simulink model "case4"  (R2024b)
settings: Solver=FixedStepAuto  StartTime=0  StopTime=1  FixedStep=1e-7  RelTol=1e-3
values from neighbouring files (symbols this model uses):
  SG_D_1_D = 0.01056    [IEEE9_case_parameters.m]    (also in case1_parameters.m; case2_parameters.m; case3_parameters.m; case4_parameters.m)
  SG_D_1_EnableSaturation = 0    [IEEE9_case_parameters.m]    (also in case1_parameters.m; case2_parameters.m; case3_parameters.m; case4_parameters.m)
  SG_D_1_f0 = 60    [IEEE9_case_parameters.m]    (also in case1_parameters.m; case2_parameters.m; case3_parameters.m; case4_parameters.m)
  SG_D_1_H = 7.5    [IEEE9_case_parameters.m]    (also in case1_parameters.m; case2_parameters.m; case3_parameters.m; case4_parameters.m)
  SG_D_1_K_A = 20    [IEEE9_case_parameters.m]    (also in case1_parameters.m; case2_parameters.m; case3_parameters.m; case4_parameters.m)
  SG_D_1_K_E = 1.000000e+1    (= 10)    [IEEE9_case_parameters.m]    (also in case1_parameters.m; case2_parameters.m; case3_parameters.m; case4_parameters.m)
  SG_D_1_K_F = 2.363    [IEEE9_case_parameters.m]    (also in case1_parameters.m; case2_parameters.m; case3_parameters.m; case4_parameters.m)
  SG_D_1_K_s = 0.5    [IEEE9_case_parameters.m]    (also in case1_parameters.m = 5; case2_parameters.m = 5; case3_parameters.m = 5; case4_parameters.m = 5)
  SG_D_1_R_a = 0.001088    [IEEE9_case_parameters.m]    (also in case1_parameters.m; case2_parameters.m; case3_parameters.m; case4_parameters.m)
  SG_D_1_S_A = 1    [IEEE9_case_parameters.m]    (also in case1_parameters.m; case2_parameters.m; case3_parameters.m; case4_parameters.m)
  SG_D_1_S_B = 0.103    [IEEE9_case_parameters.m]    (also in case1_parameters.m; case2_parameters.m; case3_parameters.m; case4_parameters.m)
  SG_D_1_S_N = 10.659857    [IEEE9_case_parameters.m]    (also in case1_parameters.m; case2_parameters.m; case3_parameters.m; case4_parameters.m)
  SG_D_1_SpeedPara = 200    [IEEE9_case_parameters.m]    (also in case1_parameters.m; case2_parameters.m; case3_parameters.m; case4_parameters.m)
  SG_D_1_T_0 = 0.720173    [IEEE9_case_parameters.m]    (also in case1_parameters.m = 0.755522; case2_parameters.m = 0.808931; case3_parameters.m = 0.869402; case4_parameters.m = 0.729316)
  SG_D_1_T_1 = 0.3    [IEEE9_case_parameters.m]    (also in case1_parameters.m; case2_parameters.m; case3_parameters.m; case4_parameters.m)
  SG_D_1_T_2 = 0.05    [IEEE9_case_parameters.m]    (also in case1_parameters.m; case2_parameters.m; case3_parameters.m; case4_parameters.m)
  SG_D_1_T_3 = 0.02    [IEEE9_case_parameters.m]    (also in case1_parameters.m; case2_parameters.m; case3_parameters.m; case4_parameters.m)
  SG_D_1_T_4 = 0.005    [IEEE9_case_parameters.m]    (also in case1_parameters.m; case2_parameters.m; case3_parameters.m; case4_parameters.m)
  SG_D_1_T_A = 0.02    [IEEE9_case_parameters.m]    (also in case1_parameters.m; case2_parameters.m; case3_parameters.m; case4_parameters.m)
  SG_D_1_T_dd = 8.000000e+0    (= 8)    [IEEE9_case_parameters.m]    (also in case1_parameters.m; case2_parameters.m; case3_parameters.m; case4_parameters.m)
  SG_D_1_T_ddd = 0.04    [IEEE9_case_parameters.m]    (also in case1_parameters.m; case2_parameters.m; case3_parameters.m; case4_parameters.m)
  SG_D_1_T_E = 0.314    [IEEE9_case_parameters.m]    (also in case1_parameters.m; case2_parameters.m; case3_parameters.m; case4_parameters.m)
  SG_D_1_T_F = 0.35    [IEEE9_case_parameters.m]    (also in case1_parameters.m; case2_parameters.m; case3_parameters.m; case4_parameters.m)
  SG_D_1_T_qd = 0.8    [IEEE9_case_parameters.m]    (also in case1_parameters.m; case2_parameters.m; case3_parameters.m; case4_parameters.m)
  SG_D_1_T_qdd = 0.02    [IEEE9_case_parameters.m]    (also in case1_parameters.m; case2_parameters.m; case3_parameters.m; case4_parameters.m)
  SG_D_1_T_speed = 0.1    [IEEE9_case_parameters.m]    (also in case1_parameters.m = 200; case2_parameters.m = 200; case3_parameters.m = 200; case4_parameters.m = 200)
  SG_D_1_T_w = 0.5    [IEEE9_case_parameters.m]    (also in case1_parameters.m; case2_parameters.m; case3_parameters.m; case4_parameters.m)
  SG_D_1_V_ref = 1.990276    [IEEE9_case_parameters.m]    (also in case1_parameters.m = 2.042296; case2_parameters.m = 2.051388; case3_parameters.m = 2.089584; case4_parameters.m = 2.01845)
  SG_D_1_w_ref = 376.991118    [IEEE9_case_parameters.m]    (also in case1_parameters.m; case2_parameters.m; case3_parameters.m; case4_parameters.m)
  SG_D_1_wb = 6.000000e+1    (= 60)    [IEEE9_case_parameters.m]    (also in case1_parameters.m; case2_parameters.m; case3_parameters.m; case4_parameters.m)
  SG_D_1_x_d = 1.9    [IEEE9_case_parameters.m]    (also in case1_parameters.m; case2_parameters.m; case3_parameters.m; case4_parameters.m)
  SG_D_1_x_dd = 0.302    [IEEE9_case_parameters.m]    (also in case1_parameters.m; case2_parameters.m; case3_parameters.m; case4_parameters.m)
  SG_D_1_x_ddd = 0.204    [IEEE9_case_parameters.m]    (also in case1_parameters.m; case2_parameters.m; case3_parameters.m; case4_parameters.m)
  SG_D_1_x_l = 0.05    [IEEE9_case_parameters.m]    (also in case1_parameters.m; case2_parameters.m; case3_parameters.m; case4_parameters.m)
  SG_D_1_x_q = 1.3    [IEEE9_case_parameters.m]    (also in case1_parameters.m; case2_parameters.m; case3_parameters.m; case4_parameters.m)
  SG_D_1_x_qd = 0.5    [IEEE9_case_parameters.m]    (also in case1_parameters.m; case2_parameters.m; case3_parameters.m; case4_parameters.m)
  SG_D_1_x_qdd = 0.3    [IEEE9_case_parameters.m]    (also in case1_parameters.m; case2_parameters.m; case3_parameters.m; case4_parameters.m)
  SG_D_2_D = 0.02    [IEEE9_case_parameters.m]    (also in case1_parameters.m; case2_parameters.m; case3_parameters.m; case4_parameters.m)
  SG_D_2_EnableSaturation = 0    [IEEE9_case_parameters.m]    (also in case1_parameters.m; case2_parameters.m; case3_parameters.m; case4_parameters.m)
  SG_D_2_f0 = 60    [IEEE9_case_parameters.m]    (also in case1_parameters.m; case2_parameters.m; case3_parameters.m; case4_parameters.m)
  SG_D_2_H = 8.000000e+0    (= 8)    [IEEE9_case_parameters.m]    (also in case1_parameters.m; case2_parameters.m; case3_parameters.m; case4_parameters.m)
  SG_D_2_K_A = 20    [IEEE9_case_parameters.m]    (also in case1_parameters.m; case2_parameters.m; case3_parameters.m; case4_parameters.m)
  SG_D_2_K_E = 1.000000e+1    (= 10)    [IEEE9_case_parameters.m]    (also in case1_parameters.m; case2_parameters.m; case3_parameters.m; case4_parameters.m)
  SG_D_2_K_F = 2.363    [IEEE9_case_parameters.m]    (also in case1_parameters.m; case2_parameters.m; case3_parameters.m; case4_parameters.m)
  SG_D_2_K_s = 0.5    [IEEE9_case_parameters.m]    (also in case1_parameters.m = 4; case2_parameters.m = 4; case3_parameters.m = 4; case4_parameters.m = 4)
  SG_D_2_R_a = 0.001088    [IEEE9_case_parameters.m]    (also in case1_parameters.m; case2_parameters.m; case3_parameters.m; case4_parameters.m)
  SG_D_2_S_A = 1    [IEEE9_case_parameters.m]    (also in case1_parameters.m; case2_parameters.m; case3_parameters.m; case4_parameters.m)
  SG_D_2_S_B = 0.103    [IEEE9_case_parameters.m]    (also in case1_parameters.m; case2_parameters.m; case3_parameters.m; case4_parameters.m)
  SG_D_2_S_N = 10.659857    [IEEE9_case_parameters.m]    (also in case1_parameters.m; case2_parameters.m; case3_parameters.m; case4_parameters.m)
  SG_D_2_SpeedPara = 200    [IEEE9_case_parameters.m]    (also in case1_parameters.m; case2_parameters.m; case3_parameters.m; case4_parameters.m)
  SG_D_2_T_0 = 1.632913    [IEEE9_case_parameters.m]    (also in case1_parameters.m = 1.632925; case2_parameters.m = 1.632915; case3_parameters.m = 1.632914; case4_parameters.m = 1.632927)
  SG_D_2_T_1 = 0.2    [IEEE9_case_parameters.m]    (also in case1_parameters.m; case2_parameters.m; case3_parameters.m; case4_parameters.m)
  SG_D_2_T_2 = 0.05    [IEEE9_case_parameters.m]    (also in case1_parameters.m; case2_parameters.m; case3_parameters.m; case4_parameters.m)
  SG_D_2_T_3 = 0.02    [IEEE9_case_parameters.m]    (also in case1_parameters.m; case2_parameters.m; case3_parameters.m; case4_parameters.m)
  SG_D_2_T_4 = 0.005    [IEEE9_case_parameters.m]    (also in case1_parameters.m; case2_parameters.m; case3_parameters.m; case4_parameters.m)
  SG_D_2_T_A = 0.02    [IEEE9_case_parameters.m]    (also in case1_parameters.m; case2_parameters.m; case3_parameters.m; case4_parameters.m)
  SG_D_2_T_dd = 7.9    [IEEE9_case_parameters.m]    (also in case1_parameters.m; case2_parameters.m; case3_parameters.m; case4_parameters.m)
  SG_D_2_T_ddd = 0.04    [IEEE9_case_parameters.m]    (also in case1_parameters.m; case2_parameters.m; case3_parameters.m; case4_parameters.m)
  SG_D_2_T_E = 0.314    [IEEE9_case_parameters.m]    (also in case1_parameters.m; case2_parameters.m; case3_parameters.m; case4_parameters.m)
  SG_D_2_T_F = 0.35    [IEEE9_case_parameters.m]    (also in case1_parameters.m; case2_parameters.m; case3_parameters.m; case4_parameters.m)
  SG_D_2_T_qd = 0.8    [IEEE9_case_parameters.m]    (also in case1_parameters.m; case2_parameters.m; case3_parameters.m; case4_parameters.m)
  SG_D_2_T_qdd = 0.015    [IEEE9_case_parameters.m]    (also in case1_parameters.m; case2_parameters.m; case3_parameters.m; case4_parameters.m)
  SG_D_2_T_speed = 0.1    [IEEE9_case_parameters.m]    (also in case1_parameters.m = 150; case2_parameters.m = 150; case3_parameters.m = 150; case4_parameters.m = 150)
  SG_D_2_T_w = 0.35    [IEEE9_case_parameters.m]    (also in case1_parameters.m; case2_parameters.m; case3_parameters.m; case4_parameters.m)
  SG_D_2_V_ref = 2.58547    [IEEE9_case_parameters.m]    (also in case1_parameters.m = 2.597896; case2_parameters.m = 2.587136; case3_parameters.m = 2.586042; case4_parameters.m = 2.599679)
  SG_D_2_w_ref = 376.991118    [IEEE9_case_parameters.m]    (also in case1_parameters.m; case2_parameters.m; case3_parameters.m; case4_parameters.m)
  SG_D_2_wb = 6.000000e+1    (= 60)    [IEEE9_case_parameters.m]    (also in case1_parameters.m; case2_parameters.m; case3_parameters.m; case4_parameters.m)
  SG_D_2_x_d = 1.8    [IEEE9_case_parameters.m]    (also in case1_parameters.m; case2_parameters.m; case3_parameters.m; case4_parameters.m)
  SG_D_2_x_dd = 0.302    [IEEE9_case_parameters.m]    (also in case1_parameters.m; case2_parameters.m; case3_parameters.m; case4_parameters.m)
  SG_D_2_x_ddd = 0.204    [IEEE9_case_parameters.m]    (also in case1_parameters.m; case2_parameters.m; case3_parameters.m; case4_parameters.m)
  SG_D_2_x_l = 0.05    [IEEE9_case_parameters.m]    (also in case1_parameters.m; case2_parameters.m; case3_parameters.m; case4_parameters.m)
  SG_D_2_x_q = 1.25    [IEEE9_case_parameters.m]    (also in case1_parameters.m; case2_parameters.m; case3_parameters.m; case4_parameters.m)
  SG_D_2_x_qd = 0.5    [IEEE9_case_parameters.m]    (also in case1_parameters.m; case2_parameters.m; case3_parameters.m; case4_parameters.m)
  SG_D_2_x_qdd = 0.3    [IEEE9_case_parameters.m]    (also in case1_parameters.m; case2_parameters.m; case3_parameters.m; case4_parameters.m)
  SG_D_3_D = 0.02    [IEEE9_case_parameters.m]    (also in case1_parameters.m; case2_parameters.m; case3_parameters.m; case4_parameters.m)
  SG_D_3_EnableSaturation = 0    [IEEE9_case_parameters.m]    (also in case1_parameters.m; case2_parameters.m; case3_parameters.m; case4_parameters.m)
  SG_D_3_f0 = 60    [IEEE9_case_parameters.m]    (also in case1_parameters.m; case2_parameters.m; case3_parameters.m; case4_parameters.m)
  SG_D_3_H = 7.7    [IEEE9_case_parameters.m]    (also in case1_parameters.m; case2_parameters.m; case3_parameters.m; case4_parameters.m)
  SG_D_3_K_A = 20    [IEEE9_case_parameters.m]    (also in case1_parameters.m; case2_parameters.m; case3_parameters.m; case4_parameters.m)
  SG_D_3_K_E = 1.000000e+1    (= 10)    [IEEE9_case_parameters.m]    (also in case1_parameters.m; case2_parameters.m; case3_parameters.m; case4_parameters.m)
  SG_D_3_K_F = 2.363    [IEEE9_case_parameters.m]    (also in case1_parameters.m; case2_parameters.m; case3_parameters.m; case4_parameters.m)
  SG_D_3_K_s = 0.2    [IEEE9_case_parameters.m]    (also in case1_parameters.m = 2; case2_parameters.m = 2; case3_parameters.m = 2; case4_parameters.m = 2)
  SG_D_3_R_a = 0.001088    [IEEE9_case_parameters.m]    (also in case1_parameters.m; case2_parameters.m; case3_parameters.m; case4_parameters.m)
  SG_D_3_S_A = 1    [IEEE9_case_parameters.m]    (also in case1_parameters.m; case2_parameters.m; case3_parameters.m; case4_parameters.m)
  SG_D_3_S_B = 0.103    [IEEE9_case_parameters.m]    (also in case1_parameters.m; case2_parameters.m; case3_parameters.m; case4_parameters.m)
  SG_D_3_S_N = 10.659857    [IEEE9_case_parameters.m]    (also in case1_parameters.m; case2_parameters.m; case3_parameters.m; case4_parameters.m)
  SG_D_3_SpeedPara = 200    [IEEE9_case_parameters.m]    (also in case1_parameters.m; case2_parameters.m; case3_parameters.m; case4_parameters.m)
  SG_D_3_T_0 = 0.850788    [IEEE9_case_parameters.m]    (also in case1_parameters.m = 0.850786; case2_parameters.m = 0.850787; case3_parameters.m; case4_parameters.m = 0.850786)
  SG_D_3_T_1 = 0.2    [IEEE9_case_parameters.m]    (also in case1_parameters.m; case2_parameters.m; case3_parameters.m; case4_parameters.m)
  SG_D_3_T_2 = 0.05    [IEEE9_case_parameters.m]    (also in case1_parameters.m; case2_parameters.m; case3_parameters.m; case4_parameters.m)
  SG_D_3_T_3 = 0.02    [IEEE9_case_parameters.m]    (also in case1_parameters.m; case2_parameters.m; case3_parameters.m; case4_parameters.m)
  SG_D_3_T_4 = 0.005    [IEEE9_case_parameters.m]    (also in case1_parameters.m; case2_parameters.m; case3_parameters.m; case4_parameters.m)
  SG_D_3_T_A = 0.02    [IEEE9_case_parameters.m]    (also in case1_parameters.m; case2_parameters.m; case3_parameters.m; case4_parameters.m)
  SG_D_3_T_dd = 8.1    [IEEE9_case_parameters.m]    (also in case1_parameters.m; case2_parameters.m; case3_parameters.m; case4_parameters.m)
  SG_D_3_T_ddd = 0.04    [IEEE9_case_parameters.m]    (also in case1_parameters.m; case2_parameters.m; case3_parameters.m; case4_parameters.m)
  SG_D_3_T_E = 0.314    [IEEE9_case_parameters.m]    (also in case1_parameters.m; case2_parameters.m; case3_parameters.m; case4_parameters.m)
  SG_D_3_T_F = 0.35    [IEEE9_case_parameters.m]    (also in case1_parameters.m; case2_parameters.m; case3_parameters.m; case4_parameters.m)
  SG_D_3_T_qd = 0.8    [IEEE9_case_parameters.m]    (also in case1_parameters.m; case2_parameters.m; case3_parameters.m; case4_parameters.m)
  SG_D_3_T_qdd = 0.015    [IEEE9_case_parameters.m]    (also in case1_parameters.m; case2_parameters.m; case3_parameters.m; case4_parameters.m)
  SG_D_3_T_speed = 0.1    [IEEE9_case_parameters.m]    (also in case1_parameters.m = 180; case2_parameters.m = 180; case3_parameters.m = 180; case4_parameters.m = 180)
  SG_D_3_T_w = 0.4    [IEEE9_case_parameters.m]    (also in case1_parameters.m; case2_parameters.m; case3_parameters.m; case4_parameters.m)
  SG_D_3_V_ref = 1.892727    [IEEE9_case_parameters.m]    (also in case1_parameters.m = 1.906439; case2_parameters.m = 1.895535; case3_parameters.m = 1.892105; case4_parameters.m = 1.906598)
  SG_D_3_w_ref = 376.991118    [IEEE9_case_parameters.m]    (also in case1_parameters.m; case2_parameters.m; case3_parameters.m; case4_parameters.m)
  SG_D_3_wb = 6.000000e+1    (= 60)    [IEEE9_case_parameters.m]    (also in case1_parameters.m; case2_parameters.m; case3_parameters.m; case4_parameters.m)
  SG_D_3_x_d = 1.85    [IEEE9_case_parameters.m]    (also in case1_parameters.m; case2_parameters.m; case3_parameters.m; case4_parameters.m)
  SG_D_3_x_dd = 0.302    [IEEE9_case_parameters.m]    (also in case1_parameters.m; case2_parameters.m; case3_parameters.m; case4_parameters.m)
  SG_D_3_x_ddd = 0.204    [IEEE9_case_parameters.m]    (also in case1_parameters.m; case2_parameters.m; case3_parameters.m; case4_parameters.m)
  SG_D_3_x_l = 0.05    [IEEE9_case_parameters.m]    (also in case1_parameters.m; case2_parameters.m; case3_parameters.m; case4_parameters.m)
  SG_D_3_x_q = 1.2    [IEEE9_case_parameters.m]    (also in case1_parameters.m; case2_parameters.m; case3_parameters.m; case4_parameters.m)
  SG_D_3_x_qd = 0.5    [IEEE9_case_parameters.m]    (also in case1_parameters.m; case2_parameters.m; case3_parameters.m; case4_parameters.m)
  SG_D_3_x_qdd = 0.3    [IEEE9_case_parameters.m]    (also in case1_parameters.m; case2_parameters.m; case3_parameters.m; case4_parameters.m)
(part 11 of 12)

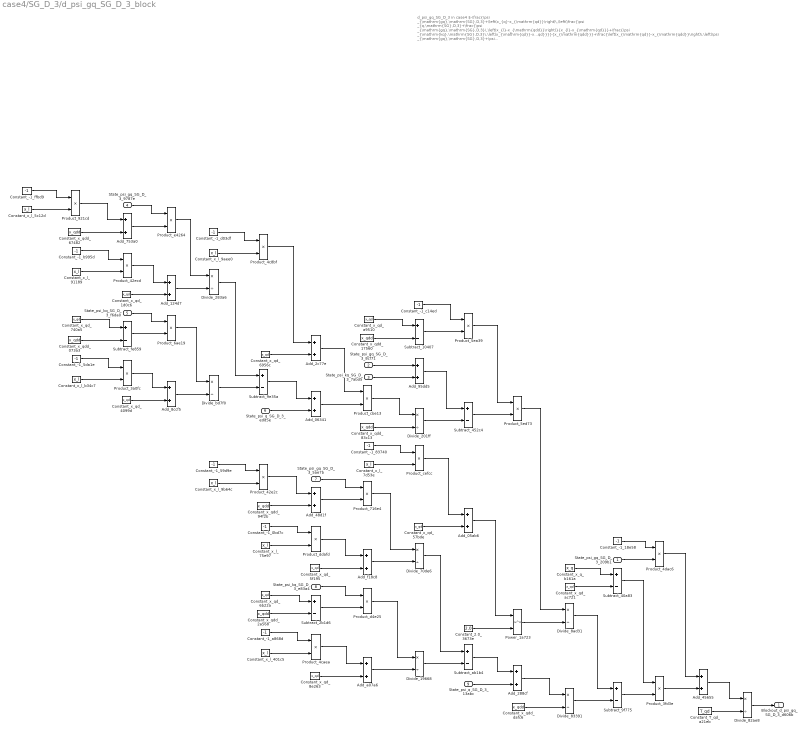
== system case4/SG_D_3/d_psi_gq_SG_D_3_block ==
  note: d_psi_gq_SG_D_3 in case4
      | $-\frac{\psi _{\mathrm{gq},\mathrm{SG},D,3}+\left(x_{q}-x_{\mathrm{qd}}\right)\,\left(\frac{\psi _{q,\mathrm{SG},D,3}+\frac{\psi _{\mathrm{gq},\mathrm{SG},D,3}\,\left(x_{l}-x_{\mathrm{qdd}}\right)}{x_{l}-x_{\mathrm{qd}}}+\frac{\psi _{\mathrm{kq},\mathrm{SG},D,3}\,\left(x_{\mathrm{qd}}-x_{\mathrm{qdd}}\right)}{x_{l}-x_{\mathrm{qd}}}}{x_{\mathrm{qdd}}}+\frac{\left(x_{\mathrm{qd}}-x_{\mathrm{qdd}}\right)\,\left(\psi _{\mathrm{gq},\mathrm{SG},D,3}+\psi _{\mathrm{kq},\mathrm{SG},D,3}+\frac{\left(x_{l}-x_{\mathrm{qd}}\right)\,\left(\psi _{q,\mathrm{SG},D,3}+\frac{\psi _{\mathrm{gq},\mathrm{SG},D,3}\,\left(x_{l}-x_{\mathrm{qdd}}\right)}{x_{l}-x_{\mathrm{qd}}}+\frac{\psi _{\mathrm{kq},\mathrm{SG},D,3}\,\left(x_{\mathrm{qd}}-x_{\mathrm{qdd}}\right)}{x_{l}-x_{\mathrm{qd}}}\right)}{x_{\mathrm{qdd}}}\right)}{{\left(x_{l}-x_{\mathrm{qd}}\right)}^2}\right)}{T_{\mathrm{qd}}}$
      | Automatically generated on 2025-10-31 19:06:33 .
  State_psi_gq_SG_D_3_209b1 : Inport
  State_psi_gq_SG_D_3_8cf71 : Inport  Port=2
  State_psi_kq_SG_D_3_7abd5 : Inport  Port=3
  State_psi_gq_SG_D_3_9787e : Inport  Port=4
  State_psi_kq_SG_D_3_f6da0 : Inport  Port=5
  State_psi_q_SG_D_3_edd5e : Inport  Port=6
  State_psi_gq_SG_D_3_5ae7b : Inport  Port=7
  State_psi_kq_SG_D_3_e83a4 : Inport  Port=8
  State_psi_q_SG_D_3_13abc : Inport  Port=9
  Add_05ab6 : Sum
  Add_06341 : Sum
  Add_124d7 : Sum
  Add_288cf : Sum
  Add_2c77e : Sum
  Add_45655 : Sum
  Add_48d1f : Sum
  Add_753a0 : Sum
  Add_8ccf5 : Sum
  Add_95dd5 : Sum
  Add_a07a6 : Sum
  Add_f18c8 : Sum
  Constant_-1_0bd7c : Constant  Value=-1
  Constant_-1_18e58 : Constant  Value=-1
  Constant_-1_59d9e : Constant  Value=-1
  Constant_-1_5da1e : Constant  Value=-1
  Constant_-1_83740 : Constant  Value=-1
  Constant_-1_a868d : Constant  Value=-1
  Constant_-1_b995d : Constant  Value=-1
  Constant_-1_c14ed : Constant  Value=-1
  Constant_-1_d03df : Constant  Value=-1
  Constant_-1_ffbd9 : Constant  Value=-1
  Constant_2.0_3673e : Constant  Value=2.0
  Constant_T_qd_a21eb : Constant  Value=T_qd
  Constant_x_l_401c5 : Constant  Value=x_l
  Constant_x_l_5c12d : Constant  Value=x_l
  Constant_x_l_75e97 : Constant  Value=x_l
  Constant_x_l_7d53e : Constant  Value=x_l
  Constant_x_l_91189 : Constant  Value=x_l
  Constant_x_l_9aee0 : Constant  Value=x_l
  Constant_x_l_9b64c : Constant  Value=x_l
  Constant_x_l_b34c7 : Constant  Value=x_l
  Constant_x_q_b161a : Constant  Value=x_q
  Constant_x_qd_1d0c6 : Constant  Value=x_qd
  Constant_x_qd_4099d : Constant  Value=x_qd
  Constant_x_qd_57bde : Constant  Value=x_qd
  Constant_x_qd_5f195 : Constant  Value=x_qd
  Constant_x_qd_6956c : Constant  Value=x_qd
  Constant_x_qd_6b22a : Constant  Value=x_qd
  Constant_x_qd_740a5 : Constant  Value=x_qd
  Constant_x_qd_8e263 : Constant  Value=x_qd
  Constant_x_qd_a9510 : Constant  Value=x_qd
  Constant_x_qd_ac721 : Constant  Value=x_qd
  Constant_x_qdd_073a3 : Constant  Value=x_qdd
  Constant_x_qdd_17560 : Constant  Value=x_qdd
  Constant_x_qdd_2a568 : Constant  Value=x_qdd
  Constant_x_qdd_67482 : Constant  Value=x_qdd
  Constant_x_qdd_83c13 : Constant  Value=x_qdd
  Constant_x_qdd_94f2b : Constant  Value=x_qdd
  Constant_x_qdd_dafc6 : Constant  Value=x_qdd
  Divide_19668 : Product  Inputs=*/
  Divide_201ff : Product  Inputs=*/
  Divide_283a6 : Product  Inputs=*/
  Divide_70de6 : Product  Inputs=*/
  Divide_82ae8 : Product  Inputs=*/
  Divide_83391 : Product  Inputs=*/
  Divide_8ad31 : Product  Inputs=*/
  Divide_bd7f0 : Product  Inputs=*/
  Power_1a723 : Math  Operator=pow
  Product_3a0fc : Product
  Product_3fd3e : Product
  Product_42e2c : Product
  Product_42ecd : Product
  Product_4c8bf : Product
  Product_4caea : Product
  Product_4dac6 : Product
  Product_5ea39 : Product
  Product_5ed73 : Product
  Product_6ae19 : Product
  Product_716e4 : Product
  Product_921cd : Product
  Product_cbe13 : Product
  Product_cefcc : Product
  Product_d4e25 : Product
  Product_ddafd : Product
  Product_e4264 : Product
  Subtract_10407 : Sum  Inputs=+-
  Subtract_2b1d6 : Sum  Inputs=+-
  Subtract_40a83 : Sum  Inputs=+-
  Subtract_452c4 : Sum  Inputs=+-
  Subtract_9e35a : Sum  Inputs=+-
  Subtract_9f775 : Sum  Inputs=+-
  Subtract_ab1b4 : Sum  Inputs=+-
  Subtract_fe859 : Sum  Inputs=+-
  Blockout_d_psi_gq_SG_D_3_d606b : Outport
  wires:
  Constant_x_l_7d53e/1 -> Product_cefcc/2
  Constant_x_qd_740a5/1 -> Subtract_fe859/1
  Add_2c77e/1 -> Product_cbe13/1
  Constant_-1_ffbd9/1 -> Product_921cd/1
  Add_753a0/1 -> Product_e4264/2
  Constant_x_qdd_073a3/1 -> Subtract_fe859/2
  Constant_x_qd_6956c/1 -> Add_2c77e/2
  Constant_x_l_5c12d/1 -> Product_921cd/2
  Constant_x_l_91189/1 -> Product_42ecd/2
  Add_a07a6/1 -> Divide_19668/2
  State_psi_kq_SG_D_3_7abd5/1 -> Add_95dd5/2
  Constant_x_qdd_67482/1 -> Add_753a0/2
  Product_921cd/1 -> Add_753a0/1
  Constant_x_qd_8e263/1 -> Add_a07a6/2
  Product_5ea39/1 -> Product_5ed73/1
  Constant_-1_59d9e/1 -> Product_42e2c/1
  Constant_-1_b995d/1 -> Product_42ecd/1
  Constant_-1_5da1e/1 -> Product_3a0fc/1
  Constant_x_l_b34c7/1 -> Product_3a0fc/2
  Constant_-1_c14ed/1 -> Product_5ea39/1
  Constant_-1_18e58/1 -> Product_4dac6/1
  State_psi_gq_SG_D_3_9787e/1 -> Product_e4264/1
  Product_42e2c/1 -> Add_48d1f/1
  Product_42ecd/1 -> Add_124d7/1
  Product_4caea/1 -> Add_a07a6/1
  Constant_x_qd_1d0c6/1 -> Add_124d7/2
  Constant_-1_0bd7c/1 -> Product_ddafd/1
  State_psi_kq_SG_D_3_f6da0/1 -> Product_6ae19/1
  Subtract_fe859/1 -> Product_6ae19/2
  Product_3a0fc/1 -> Add_8ccf5/1
  Add_48d1f/1 -> Product_716e4/2
  Add_124d7/1 -> Divide_283a6/2
  Constant_x_qd_4099d/1 -> Add_8ccf5/2
  Product_e4264/1 -> Divide_283a6/1
  Constant_T_qd_a21eb/1 -> Divide_82ae8/2
  Product_ddafd/1 -> Add_f18c8/1
  Product_6ae19/1 -> Divide_bd7f0/1
  Product_d4e25/1 -> Divide_19668/1
  Add_8ccf5/1 -> Divide_bd7f0/2
  Constant_-1_d03df/1 -> Product_4c8bf/1
  Constant_x_qdd_83c13/1 -> Divide_201ff/2
  Constant_x_l_9aee0/1 -> Product_4c8bf/2
  Divide_283a6/1 -> Subtract_9e35a/1
  Constant_x_qd_ac721/1 -> Subtract_40a83/2
  Add_f18c8/1 -> Divide_70de6/2
  Divide_bd7f0/1 -> Subtract_9e35a/2
  Constant_x_l_9b64c/1 -> Product_42e2c/2
  Product_4c8bf/1 -> Add_2c77e/1
  Constant_-1_83740/1 -> Product_cefcc/1
  Constant_x_l_75e97/1 -> Product_ddafd/2
  Subtract_9e35a/1 -> Add_06341/1
  State_psi_q_SG_D_3_edd5e/1 -> Add_06341/2
  Constant_-1_a868d/1 -> Product_4caea/1
  Constant_x_qdd_94f2b/1 -> Add_48d1f/2
  Constant_x_qd_6b22a/1 -> Subtract_2b1d6/1
  Constant_x_qdd_2a568/1 -> Subtract_2b1d6/2
  Constant_x_l_401c5/1 -> Product_4caea/2
  Add_06341/1 -> Product_cbe13/2
  Constant_x_qdd_17560/1 -> Subtract_10407/2
  State_psi_gq_SG_D_3_5ae7b/1 -> Product_716e4/1
  Constant_x_qd_5f195/1 -> Add_f18c8/2
  Divide_8ad31/1 -> Subtract_9f775/1
  State_psi_kq_SG_D_3_e83a4/1 -> Product_d4e25/1
  Subtract_2b1d6/1 -> Product_d4e25/2
  Constant_x_qd_a9510/1 -> Subtract_10407/1
  State_psi_gq_SG_D_3_8cf71/1 -> Add_95dd5/1
  Product_cbe13/1 -> Divide_201ff/1
  Product_716e4/1 -> Divide_70de6/1
  Subtract_10407/1 -> Product_5ea39/2
  Add_95dd5/1 -> Subtract_452c4/1
  Divide_201ff/1 -> Subtract_452c4/2
  Product_cefcc/1 -> Add_05ab6/1
  Constant_x_qd_57bde/1 -> Add_05ab6/2
  Divide_70de6/1 -> Subtract_ab1b4/1
  Divide_19668/1 -> Subtract_ab1b4/2
  Subtract_452c4/1 -> Product_5ed73/2
  Add_05ab6/1 -> Power_1a723/1
  Constant_2.0_3673e/1 -> Power_1a723/2
  Subtract_ab1b4/1 -> Add_288cf/1
  State_psi_q_SG_D_3_13abc/1 -> Add_288cf/2
  Product_5ed73/1 -> Divide_8ad31/1
  Power_1a723/1 -> Divide_8ad31/2
  Add_288cf/1 -> Divide_83391/1
  Constant_x_qdd_dafc6/1 -> Divide_83391/2
  Constant_x_q_b161a/1 -> Subtract_40a83/1
  Divide_83391/1 -> Subtract_9f775/2
  State_psi_gq_SG_D_3_209b1/1 -> Product_4dac6/2
  Subtract_40a83/1 -> Product_3fd3e/1
  Subtract_9f775/1 -> Product_3fd3e/2
  Product_4dac6/1 -> Add_45655/1
  Product_3fd3e/1 -> Add_45655/2
  Add_45655/1 -> Divide_82ae8/1
  Divide_82ae8/1 -> Blockout_d_psi_gq_SG_D_3_d606b/1

== system case4/SG_D_3/d_psi_kq_SG_D_3_block ==
  note: d_psi_kq_SG_D_3 in case4
      | $-\frac{\psi _{\mathrm{gq},\mathrm{SG},D,3}+\psi _{\mathrm{kq},\mathrm{SG},D,3}+\frac{\left(x_{l}-x_{\mathrm{qd}}\right)\,\left(\psi _{q,\mathrm{SG},D,3}+\frac{\psi _{\mathrm{gq},\mathrm{SG},D,3}\,\left(x_{l}-x_{\mathrm{qdd}}\right)}{x_{l}-x_{\mathrm{qd}}}+\frac{\psi _{\mathrm{kq},\mathrm{SG},D,3}\,\left(x_{\mathrm{qd}}-x_{\mathrm{qdd}}\right)}{x_{l}-x_{\mathrm{qd}}}\right)}{x_{\mathrm{qdd}}}}{T_{\mathrm{qdd}}}$
      | Automatically generated on 2025-10-31 19:06:36 .
  State_psi_gq_SG_D_3_8599d : Inport
  State_psi_kq_SG_D_3_56f6b : Inport  Port=2
  State_psi_gq_SG_D_3_442bf : Inport  Port=3
  State_psi_kq_SG_D_3_5af45 : Inport  Port=4
  State_psi_q_SG_D_3_8b826 : Inport  Port=5
  Add_6a84b : Sum
  Add_7ec4b : Sum
  Add_86454 : Sum
  Add_880a1 : Sum
  Add_bfbab : Sum
  Add_cfc57 : Sum
  Constant_-1_08f4c : Constant  Value=-1
  Constant_-1_3eac4 : Constant  Value=-1
  Constant_-1_773e8 : Constant  Value=-1
  Constant_-1_9a346 : Constant  Value=-1
  Constant_-1_f5dc2 : Constant  Value=-1
  Constant_T_qdd_de64c : Constant  Value=T_qdd
  Constant_x_l_58b40 : Constant  Value=x_l
  Constant_x_l_5aa6e : Constant  Value=x_l
  Constant_x_l_9719e : Constant  Value=x_l
  Constant_x_l_b944f : Constant  Value=x_l
  Constant_x_qd_1e917 : Constant  Value=x_qd
  Constant_x_qd_40938 : Constant  Value=x_qd
  Constant_x_qd_9dafc : Constant  Value=x_qd
  Constant_x_qd_ffde1 : Constant  Value=x_qd
  Constant_x_qdd_3a31b : Constant  Value=x_qdd
  Constant_x_qdd_c24c8 : Constant  Value=x_qdd
  Constant_x_qdd_d4eaf : Constant  Value=x_qdd
  Divide_4b065 : Product  Inputs=*/
  Divide_6a055 : Product  Inputs=*/
  Divide_8d63f : Product  Inputs=*/
  Divide_a8841 : Product  Inputs=*/
  Product_0564a : Product
  Product_15596 : Product
  Product_3b6ea : Product
  Product_6a8c1 : Product
  Product_806dc : Product
  Product_9c4e9 : Product
  Product_b860e : Product
  Product_d2c3a : Product
  Subtract_3bca2 : Sum  Inputs=+-
  Subtract_5b7c8 : Sum  Inputs=+-
  Subtract_9f6fc : Sum  Inputs=+-
  Blockout_d_psi_kq_SG_D_3_86686 : Outport
  wires:
  State_psi_q_SG_D_3_8b826/1 -> Add_cfc57/2
  Constant_-1_773e8/1 -> Product_9c4e9/1
  Constant_-1_9a346/1 -> Product_3b6ea/1
  Constant_-1_3eac4/1 -> Product_b860e/1
  Constant_x_l_b944f/1 -> Product_9c4e9/2
  Constant_x_qdd_d4eaf/1 -> Add_6a84b/2
  Product_15596/1 -> Add_bfbab/1
  Constant_x_l_5aa6e/1 -> Product_3b6ea/2
  Constant_x_qd_40938/1 -> Subtract_9f6fc/1
  Product_3b6ea/1 -> Add_6a84b/1
  Constant_x_l_9719e/1 -> Product_0564a/2
  Constant_x_qdd_3a31b/1 -> Subtract_9f6fc/2
  Constant_-1_f5dc2/1 -> Product_15596/1
  Constant_x_l_58b40/1 -> Product_15596/2
  State_psi_gq_SG_D_3_442bf/1 -> Product_6a8c1/1
  Add_6a84b/1 -> Product_6a8c1/2
  Add_cfc57/1 -> Product_806dc/2
  Product_9c4e9/1 -> Add_7ec4b/1
  Constant_x_qd_9dafc/1 -> Add_7ec4b/2
  State_psi_kq_SG_D_3_5af45/1 -> Product_d2c3a/1
  Subtract_9f6fc/1 -> Product_d2c3a/2
  Add_7ec4b/1 -> Divide_6a055/2
  Constant_x_qd_1e917/1 -> Add_bfbab/2
  Product_6a8c1/1 -> Divide_6a055/1
  Product_d2c3a/1 -> Divide_4b065/1
  Add_bfbab/1 -> Divide_4b065/2
  Constant_-1_08f4c/1 -> Product_0564a/1
  Divide_6a055/1 -> Subtract_3bca2/1
  Add_86454/1 -> Divide_8d63f/1
  Divide_4b065/1 -> Subtract_3bca2/2
  Divide_8d63f/1 -> Blockout_d_psi_kq_SG_D_3_86686/1
  Product_0564a/1 -> Add_880a1/1
  Constant_x_qd_ffde1/1 -> Add_880a1/2
  Subtract_3bca2/1 -> Add_cfc57/1
  State_psi_gq_SG_D_3_8599d/1 -> Product_b860e/2
  Add_880a1/1 -> Product_806dc/1
  Constant_T_qdd_de64c/1 -> Divide_8d63f/2
  Product_b860e/1 -> Subtract_5b7c8/1
  State_psi_kq_SG_D_3_56f6b/1 -> Subtract_5b7c8/2
  Product_806dc/1 -> Divide_a8841/1
  Constant_x_qdd_c24c8/1 -> Divide_a8841/2
  Subtract_5b7c8/1 -> Add_86454/1
  Divide_a8841/1 -> Add_86454/2

== system case4/SG_D_3/d_psi_q_SG_D_3_block ==
  note: d_psi_q_SG_D_3 in case4
      | $2\,\pi \,f_{0}\,\left(v_{d,\mathrm{SG},D,3}\,\cos\left(\theta _{\mathrm{SG},D,3}\right)+v_{q,\mathrm{SG},D,3}\,\sin\left(\theta _{\mathrm{SG},D,3}\right)-\frac{R_{a}\,\left(\psi _{q,\mathrm{SG},D,3}+\frac{\psi _{\mathrm{gq},\mathrm{SG},D,3}\,\left(x_{l}-x_{\mathrm{qdd}}\right)}{x_{l}-x_{\mathrm{qd}}}+\frac{\psi _{\mathrm{kq},\mathrm{SG},D,3}\,\left(x_{\mathrm{qd}}-x_{\mathrm{qdd}}\right)}{x_{l}-x_{\mathrm{qd}}}\right)}{x_{\mathrm{qdd}}}-\frac{\psi _{d,\mathrm{SG},D,3}\,w_{\mathrm{SG},D,3}}{2\,f_{0}\,\pi }\right)$
      | Automatically generated on 2025-10-31 19:06:20 .
  State_psi_gq_SG_D_3_4bbcf : Inport
  State_psi_kq_SG_D_3_07912 : Inport  Port=2
  State_psi_q_SG_D_3_50e34 : Inport  Port=3
  Input_v_d_SG_D_3_64638 : Inport  Port=4
  State_theta_SG_D_3_91f0b : Inport  Port=5
  Input_v_q_SG_D_3_99a28 : Inport  Port=6
  State_theta_SG_D_3_8654b : Inport  Port=7
  State_psi_d_SG_D_3_31b80 : Inport  Port=8
  State_w_SG_D_3_e8c7b : Inport  Port=9
  Add_55a1e : Sum
  Add_68a51 : Sum
  Add_86217 : Sum
  Add_9dd7c : Sum
  Add_ccee4 : Sum
  Constant_-1_5b7d1 : Constant  Value=-1
  Constant_-1_ab0cd : Constant  Value=-1
  Constant_-1_f9165 : Constant  Value=-1
  Constant_-2.0_72dce : Constant  Value=-2.0
  Constant_2.0_03fb8 : Constant  Value=2.0
  Constant_R_a_e2632 : Constant  Value=R_a
  Constant_f0_1b7bd : Constant  Value=f0
  Constant_f0_6aa71 : Constant  Value=f0
  Constant_pi_2ca87 : Constant  Value=pi
  Constant_pi_88f4f : Constant  Value=pi
  Constant_x_l_06ff6 : Constant  Value=x_l
  Constant_x_l_4b09f : Constant  Value=x_l
  Constant_x_l_e78f6 : Constant  Value=x_l
  Constant_x_qd_1df14 : Constant  Value=x_qd
  Constant_x_qd_9aa9b : Constant  Value=x_qd
  Constant_x_qd_c28c4 : Constant  Value=x_qd
  Constant_x_qdd_4d22a : Constant  Value=x_qdd
  Constant_x_qdd_c25c2 : Constant  Value=x_qdd
  Constant_x_qdd_cd72f : Constant  Value=x_qdd
  Divide_2a95f : Product  Inputs=*/
  Divide_c93f2 : Product  Inputs=*/
  Divide_eec2e : Product  Inputs=*/
  Divide_f611a : Product  Inputs=*/
  MathFunc_cos_987f6 : Trigonometry  Operator=cos
  MathFunc_sin_56b54 : Trigonometry
  Product_4a20d : Product
  Product_6a9c1 : Product
  Product_6f205 : Product
  Product_77700 : Product
  Product_810f2 : Product
  Product_94db4 : Product
  Product_a6da9 : Product
  Product_a864b : Product
  Product_bab32 : Product
  Product_c0eb1 : Product
  Product_c6203 : Product
  Product_ccbc6 : Product
  Product_ebed2 : Product
  Product_ed576 : Product
  Subtract_07f7a : Sum  Inputs=+-
  Subtract_69425 : Sum  Inputs=+-
  Subtract_7e7b9 : Sum  Inputs=+-
  Subtract_93d2e : Sum  Inputs=+-
  Blockout_d_psi_q_SG_D_3_12ce6 : Outport
  wires:
  Constant_x_qd_9aa9b/1 -> Subtract_93d2e/1
  Constant_pi_88f4f/1 -> Product_ccbc6/2
  Product_ed576/1 -> Divide_f611a/1
  Constant_x_l_4b09f/1 -> Product_ebed2/2
  Constant_f0_1b7bd/1 -> Product_a864b/2
  State_w_SG_D_3_e8c7b/1 -> Product_c0eb1/2
  Constant_-1_f9165/1 -> Product_77700/1
  Constant_x_qdd_cd72f/1 -> Add_68a51/2
  Input_v_d_SG_D_3_64638/1 -> Product_94db4/1
  Constant_x_qdd_c25c2/1 -> Subtract_93d2e/2
  Constant_x_l_06ff6/1 -> Product_77700/2
  Divide_2a95f/1 -> Add_55a1e/2
  Product_77700/1 -> Add_68a51/1
  Constant_2.0_03fb8/1 -> Product_ccbc6/1
  Add_9dd7c/1 -> Product_ed576/2
  Constant_-1_5b7d1/1 -> Product_ebed2/1
  Constant_x_qd_1df14/1 -> Add_86217/2
  Constant_-1_ab0cd/1 -> Product_810f2/1
  Subtract_07f7a/1 -> Subtract_7e7b9/1
  Constant_x_l_e78f6/1 -> Product_810f2/2
  Subtract_7e7b9/1 -> Add_55a1e/1
  Constant_f0_6aa71/1 -> Product_6a9c1/2
  State_theta_SG_D_3_8654b/1 -> MathFunc_sin_56b54/1
  Constant_x_qd_c28c4/1 -> Add_ccee4/2
  State_psi_gq_SG_D_3_4bbcf/1 -> Product_c6203/1
  Add_68a51/1 -> Product_c6203/2
  Product_ccbc6/1 -> Product_6a9c1/1
  Product_ebed2/1 -> Add_ccee4/1
  State_psi_kq_SG_D_3_07912/1 -> Product_a6da9/1
  Subtract_93d2e/1 -> Product_a6da9/2
  Product_810f2/1 -> Add_86217/1
  MathFunc_sin_56b54/1 -> Product_bab32/2
  Product_c6203/1 -> Divide_eec2e/1
  Product_6a9c1/1 -> Divide_2a95f/2
  Add_ccee4/1 -> Divide_eec2e/2
  Product_a6da9/1 -> Divide_c93f2/1
  Add_86217/1 -> Divide_c93f2/2
  Input_v_q_SG_D_3_99a28/1 -> Product_bab32/1
  Divide_eec2e/1 -> Subtract_69425/1
  Subtract_69425/1 -> Add_9dd7c/1
  Divide_c93f2/1 -> Subtract_69425/2
  Divide_f611a/1 -> Subtract_07f7a/1
  State_psi_q_SG_D_3_50e34/1 -> Add_9dd7c/2
  Product_bab32/1 -> Subtract_7e7b9/2
  Constant_R_a_e2632/1 -> Product_ed576/1
  State_theta_SG_D_3_91f0b/1 -> MathFunc_cos_987f6/1
  Constant_x_qdd_4d22a/1 -> Divide_f611a/2
  MathFunc_cos_987f6/1 -> Product_94db4/2
  Constant_-2.0_72dce/1 -> Product_4a20d/1
  Product_94db4/1 -> Subtract_07f7a/2
  State_psi_d_SG_D_3_31b80/1 -> Product_c0eb1/1
  Constant_pi_2ca87/1 -> Product_4a20d/2
  Product_c0eb1/1 -> Divide_2a95f/1
  Product_4a20d/1 -> Product_a864b/1
  Product_a864b/1 -> Product_6f205/1
  Add_55a1e/1 -> Product_6f205/2
  Product_6f205/1 -> Blockout_d_psi_q_SG_D_3_12ce6/1

== system case4/SG_D_3/d_theta_SG_D_3_block ==
  note: d_theta_SG_D_3 in case4
      | $w_{\mathrm{SG},D,3}-2\,\pi \,f_{0}$
      | Automatically generated on 2025-10-31 19:06:43 .
  State_w_SG_D_3_e7367 : Inport
  Add_f93ba : Sum
  Constant_-2.0_92430 : Constant  Value=-2.0
  Constant_f0_4a707 : Constant  Value=f0
  Constant_pi_37e55 : Constant  Value=pi
  Product_4b160 : Product
  Product_5147a : Product
  Blockout_d_theta_SG_D_3_449e6 : Outport
  wires:
  Constant_-2.0_92430/1 -> Product_4b160/1
  Constant_pi_37e55/1 -> Product_4b160/2
  State_w_SG_D_3_e7367/1 -> Add_f93ba/2
  Product_4b160/1 -> Product_5147a/1
  Constant_f0_4a707/1 -> Product_5147a/2
  Product_5147a/1 -> Add_f93ba/1
  Add_f93ba/1 -> Blockout_d_theta_SG_D_3_449e6/1

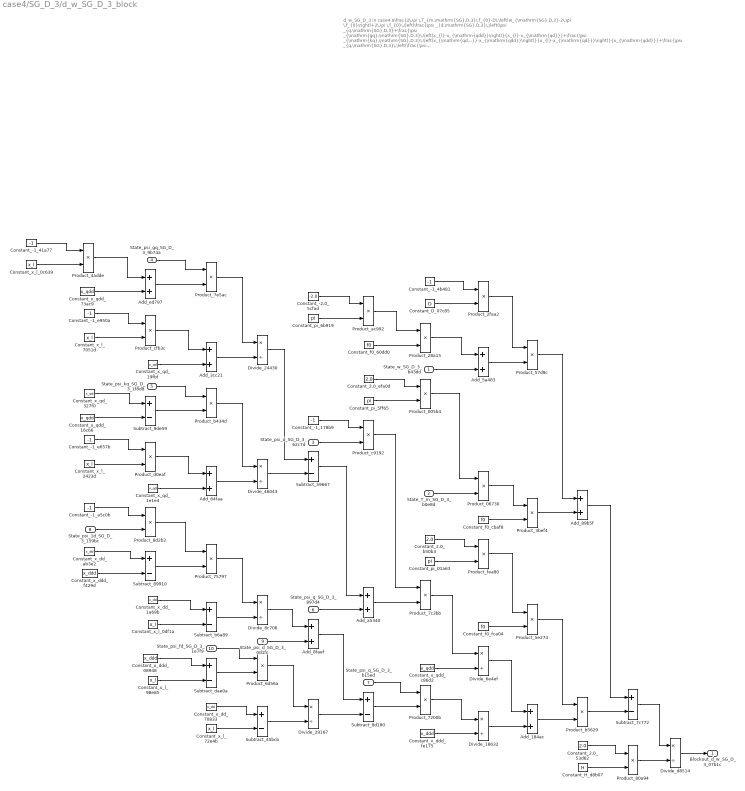
== system case4/SG_D_3/d_w_SG_D_3_block ==
  note: d_w_SG_D_3 in case4
      | $\frac{2\,\pi \,T_{m,\mathrm{SG},D,3}\,f_{0}-D\,\left(w_{\mathrm{SG},D,3}-2\,\pi \,f_{0}\right)+2\,\pi \,f_{0}\,\left(\frac{\psi _{d,\mathrm{SG},D,3}\,\left(\psi _{q,\mathrm{SG},D,3}+\frac{\psi _{\mathrm{gq},\mathrm{SG},D,3}\,\left(x_{l}-x_{\mathrm{qdd}}\right)}{x_{l}-x_{\mathrm{qd}}}+\frac{\psi _{\mathrm{kq},\mathrm{SG},D,3}\,\left(x_{\mathrm{qd}}-x_{\mathrm{qdd}}\right)}{x_{l}-x_{\mathrm{qd}}}\right)}{x_{\mathrm{qdd}}}+\frac{\psi _{q,\mathrm{SG},D,3}\,\left(\frac{\psi _{\mathrm{1d},\mathrm{SG},D,3}\,\left(x_{\mathrm{dd}}-x_{\mathrm{ddd}}\right)}{x_{\mathrm{dd}}-x_{l}}-\psi _{d,\mathrm{SG},D,3}+\frac{\psi _{\mathrm{fd},\mathrm{SG},D,3}\,\left(x_{\mathrm{ddd}}-x_{l}\right)}{x_{\mathrm{dd}}-x_{l}}\right)}{x_{\mathrm{ddd}}}\right)}{2\,H}$
      | Automatically generated on 2025-10-31 19:06:42 .
  State_w_SG_D_3_b43dd : Inport
  State_T_m_SG_D_3_b0e8d : Inport  Port=2
  State_psi_d_SG_D_3_62c7d : Inport  Port=3
  State_psi_gq_SG_D_3_9b74a : Inport  Port=4
  State_psi_kq_SG_D_3_1f8d8 : Inport  Port=5
  State_psi_q_SG_D_3_897d4 : Inport  Port=6
  State_psi_q_SG_D_3_b15ed : Inport  Port=7
  State_psi_1d_SG_D_3_159bc : Inport  Port=8
  State_psi_d_SG_D_3_0d1fc : Inport  Port=9
  State_psi_fd_SG_D_3_1e7f9 : Inport  Port=10
  Add_184ac : Sum
  Add_3cc21 : Sum
  Add_5a483 : Sum
  Add_64faa : Sum
  Add_89b5f : Sum
  Add_8faef : Sum
  Add_a5340 : Sum
  Add_ed797 : Sum
  Constant_-1_178b9 : Constant  Value=-1
  Constant_-1_41a77 : Constant  Value=-1
  Constant_-1_4b481 : Constant  Value=-1
  Constant_-1_a5c0b : Constant  Value=-1
  Constant_-1_e657b : Constant  Value=-1
  Constant_-1_e950a : Constant  Value=-1
  Constant_-2.0_5cfad : Constant  Value=-2.0
  Constant_2.0_53d62 : Constant  Value=2.0
  Constant_2.0_b50b3 : Constant  Value=2.0
  Constant_2.0_efa0d : Constant  Value=2.0
  Constant_D_07c85 : Constant  Value=D
  Constant_H_d8b07 : Constant  Value=H
  Constant_f0_60dd0 : Constant  Value=f0
  Constant_f0_cbaf8 : Constant  Value=f0
  Constant_f0_fca04 : Constant  Value=f0
  Constant_pi_01a63 : Constant  Value=pi
  Constant_pi_5ff65 : Constant  Value=pi
  Constant_pi_6b919 : Constant  Value=pi
  Constant_x_dd_1a69b : Constant  Value=x_dd
  Constant_x_dd_70833 : Constant  Value=x_dd
  Constant_x_dd_ab3e2 : Constant  Value=x_dd
  Constant_x_ddd_08948 : Constant  Value=x_ddd
  Constant_x_ddd_f429d : Constant  Value=x_ddd
  Constant_x_ddd_fe175 : Constant  Value=x_ddd
  Constant_x_l_0c639 : Constant  Value=x_l
  Constant_x_l_0df1a : Constant  Value=x_l
  Constant_x_l_2423d : Constant  Value=x_l
  Constant_x_l_7051d : Constant  Value=x_l
  Constant_x_l_72e4b : Constant  Value=x_l
  Constant_x_l_98e85 : Constant  Value=x_l
  Constant_x_qd_19fbf : Constant  Value=x_qd
  Constant_x_qd_1e1e4 : Constant  Value=x_qd
  Constant_x_qd_327f0 : Constant  Value=x_qd
  Constant_x_qdd_16c66 : Constant  Value=x_qdd
  Constant_x_qdd_73ac9 : Constant  Value=x_qdd
  Constant_x_qdd_c86d2 : Constant  Value=x_qdd
  Divide_{18632,24430,29167,46043} (4 alike) : Product  Inputs=*/
  Divide_6e4ef : Product  Inputs=*/
  Divide_8c706 : Product  Inputs=*/
  Divide_d8514 : Product  Inputs=*/
  Product_005b4 : Product
  Product_06730 : Product
  Product_28a15 : Product
  Product_2faa2 : Product
  Product_3bef4 : Product
  Product_4adde : Product
  Product_57d9c : Product
  Product_5e274 : Product
  Product_6d56a : Product
  Product_7200b : Product
  Product_75797 : Product
  Product_7c3bb : Product
  Product_7e5ac : Product
  Product_80a94 : Product
  Product_8d2b2 : Product
  Product_ac992 : Product
  Product_b434d : Product
  Product_b5629 : Product
  Product_c9192 : Product
  Product_cfb3c : Product
  Product_d0eaf : Product
  Product_fea80 : Product
  Subtract_45bcb : Sum  Inputs=+-
  Subtract_59667 : Sum  Inputs=+-
  Subtract_7c772 : Sum  Inputs=+-
  Subtract_89910 : Sum  Inputs=+-
  Subtract_8d180 : Sum  Inputs=+-
  Subtract_9de59 : Sum  Inputs=+-
  Subtract_b6a89 : Sum  Inputs=+-
  Subtract_dae0a : Sum  Inputs=+-
  Blockout_d_w_SG_D_3_07b1c : Outport
  wires:
  Constant_x_qd_327f0/1 -> Subtract_9de59/1
  Subtract_89910/1 -> Product_75797/2
  Subtract_7c772/1 -> Divide_d8514/1
  Constant_-1_41a77/1 -> Product_4adde/1
  Add_ed797/1 -> Product_7e5ac/2
  Constant_x_qdd_16c66/1 -> Subtract_9de59/2
  Subtract_dae0a/1 -> Product_6d56a/2
  Constant_x_l_0c639/1 -> Product_4adde/2
  State_psi_d_SG_D_3_0d1fc/1 -> Add_8faef/2
  Add_3cc21/1 -> Divide_24430/2
  Constant_x_dd_1a69b/1 -> Subtract_b6a89/1
  Constant_x_l_7051d/1 -> Product_cfb3c/2
  Constant_-1_4b481/1 -> Product_2faa2/1
  Divide_29167/1 -> Subtract_8d180/2
  Constant_x_ddd_f429d/1 -> Subtract_89910/2
  Constant_x_qdd_73ac9/1 -> Add_ed797/2
  Constant_pi_5ff65/1 -> Product_005b4/2
  Product_4adde/1 -> Add_ed797/1
  Constant_-2.0_5cfad/1 -> Product_ac992/1
  Constant_-1_e950a/1 -> Product_cfb3c/1
  Constant_2.0_b50b3/1 -> Product_fea80/1
  Product_ac992/1 -> Product_28a15/1
  Constant_-1_e657b/1 -> Product_d0eaf/1
  Subtract_59667/1 -> Add_a5340/1
  Constant_x_l_2423d/1 -> Product_d0eaf/2
  Constant_x_l_98e85/1 -> Subtract_dae0a/2
  Constant_-1_a5c0b/1 -> Product_8d2b2/1
  State_psi_1d_SG_D_3_159bc/1 -> Product_8d2b2/2
  Constant_x_dd_ab3e2/1 -> Subtract_89910/1
  Product_8d2b2/1 -> Product_75797/1
  State_psi_gq_SG_D_3_9b74a/1 -> Product_7e5ac/1
  Constant_x_qd_19fbf/1 -> Add_3cc21/2
  Product_cfb3c/1 -> Add_3cc21/1
  State_psi_kq_SG_D_3_1f8d8/1 -> Product_b434d/1
  Subtract_9de59/1 -> Product_b434d/2
  Product_fea80/1 -> Product_5e274/1
  Product_28a15/1 -> Add_5a483/1
  Product_d0eaf/1 -> Add_64faa/1
  State_psi_q_SG_D_3_b15ed/1 -> Product_7200b/1
  Constant_x_qd_1e1e4/1 -> Add_64faa/2
  Constant_x_l_0df1a/1 -> Subtract_b6a89/2
  Constant_x_ddd_08948/1 -> Subtract_dae0a/1
  Constant_x_l_72e4b/1 -> Subtract_45bcb/2
  Product_7e5ac/1 -> Divide_24430/1
  Product_b434d/1 -> Divide_46043/1
  Add_64faa/1 -> Divide_46043/2
  Product_75797/1 -> Divide_8c706/1
  Subtract_b6a89/1 -> Divide_8c706/2
  Constant_2.0_efa0d/1 -> Product_005b4/1
  State_psi_fd_SG_D_3_1e7f9/1 -> Product_6d56a/1
  Constant_x_dd_70833/1 -> Subtract_45bcb/1
  Divide_24430/1 -> Subtract_59667/1
  Product_6d56a/1 -> Divide_29167/1
  Divide_46043/1 -> Subtract_59667/2
  Divide_8c706/1 -> Add_8faef/1
  Product_b5629/1 -> Subtract_7c772/2
  Subtract_45bcb/1 -> Divide_29167/2
  Constant_pi_6b919/1 -> Product_ac992/2
  Constant_pi_01a63/1 -> Product_fea80/2
  Constant_-1_178b9/1 -> Product_c9192/1
  State_psi_d_SG_D_3_62c7d/1 -> Product_c9192/2
  State_psi_q_SG_D_3_897d4/1 -> Add_a5340/2
  Add_8faef/1 -> Subtract_8d180/1
  Constant_f0_60dd0/1 -> Product_28a15/2
  Product_c9192/1 -> Product_7c3bb/1
  Add_a5340/1 -> Product_7c3bb/2
  Subtract_8d180/1 -> Product_7200b/2
  Constant_D_07c85/1 -> Product_2faa2/2
  State_w_SG_D_3_b43dd/1 -> Add_5a483/2
  Product_005b4/1 -> Product_06730/1
  State_T_m_SG_D_3_b0e8d/1 -> Product_06730/2
  Product_7c3bb/1 -> Divide_6e4ef/1
  Constant_x_qdd_c86d2/1 -> Divide_6e4ef/2
  Product_7200b/1 -> Divide_18632/1
  Constant_x_ddd_fe175/1 -> Divide_18632/2
  Product_2faa2/1 -> Product_57d9c/1
  Add_5a483/1 -> Product_57d9c/2
  Product_06730/1 -> Product_3bef4/1
  Constant_f0_cbaf8/1 -> Product_3bef4/2
  Constant_f0_fca04/1 -> Product_5e274/2
  Divide_6e4ef/1 -> Add_184ac/1
  Divide_18632/1 -> Add_184ac/2
  Product_57d9c/1 -> Add_89b5f/1
  Product_3bef4/1 -> Add_89b5f/2
  Product_5e274/1 -> Product_b5629/1
  Add_184ac/1 -> Product_b5629/2
  Add_89b5f/1 -> Subtract_7c772/1
  Constant_2.0_53d62/1 -> Product_80a94/1
  Constant_H_d8b07/1 -> Product_80a94/2
  Product_80a94/1 -> Divide_d8514/2
  Divide_d8514/1 -> Blockout_d_w_SG_D_3_07b1c/1

== system case4/SG_D_3/i_d_SG_D_3_block ==
  note: i_d_SG_D_3 in case4
      | $\frac{\sin\left(\theta _{\mathrm{SG},D,3}\right)\,\left(\frac{\psi _{\mathrm{1d},\mathrm{SG},D,3}\,\left(x_{\mathrm{dd}}-x_{\mathrm{ddd}}\right)}{x_{\mathrm{dd}}-x_{l}}-\psi _{d,\mathrm{SG},D,3}+\frac{\psi _{\mathrm{fd},\mathrm{SG},D,3}\,\left(x_{\mathrm{ddd}}-x_{l}\right)}{x_{\mathrm{dd}}-x_{l}}\right)}{x_{\mathrm{ddd}}}-\frac{\cos\left(\theta _{\mathrm{SG},D,3}\right)\,\left(\psi _{q,\mathrm{SG},D,3}+\frac{\psi _{\mathrm{gq},\mathrm{SG},D,3}\,\left(x_{l}-x_{\mathrm{qdd}}\right)}{x_{l}-x_{\mathrm{qd}}}+\frac{\psi _{\mathrm{kq},\mathrm{SG},D,3}\,\left(x_{\mathrm{qd}}-x_{\mathrm{qdd}}\right)}{x_{l}-x_{\mathrm{qd}}}\right)}{x_{\mathrm{qdd}}}$
      | Automatically generated on 2025-10-31 19:07:02 .
  State_psi_gq_SG_D_3_033c6 : Inport
  State_psi_kq_SG_D_3_67dcb : Inport  Port=2
  State_psi_q_SG_D_3_1df08 : Inport  Port=3
  State_theta_SG_D_3_0b2a8 : Inport  Port=4
  State_psi_1d_SG_D_3_e063f : Inport  Port=5
  State_psi_d_SG_D_3_e7225 : Inport  Port=6
  State_psi_fd_SG_D_3_2fd40 : Inport  Port=7
  State_theta_SG_D_3_6b34c : Inport  Port=8
  Add_8a214 : Sum
  Add_92cd6 : Sum
  Add_a17fd : Sum
  Add_dfa2f : Sum
  Add_ea115 : Sum
  Constant_-1_23574 : Constant  Value=-1
  Constant_-1_687e4 : Constant  Value=-1
  Constant_-1_6883c : Constant  Value=-1
  Constant_-1_75f1e : Constant  Value=-1
  Constant_-1_cf294 : Constant  Value=-1
  Constant_x_dd_7bc64 : Constant  Value=x_dd
  Constant_x_dd_b5763 : Constant  Value=x_dd
  Constant_x_dd_eff09 : Constant  Value=x_dd
  Constant_x_ddd_23990 : Constant  Value=x_ddd
  Constant_x_ddd_259c8 : Constant  Value=x_ddd
  Constant_x_ddd_9648b : Constant  Value=x_ddd
  Constant_x_l_4d31d : Constant  Value=x_l
  Constant_x_l_6f196 : Constant  Value=x_l
  Constant_x_l_79434 : Constant  Value=x_l
  Constant_x_l_9e4c3 : Constant  Value=x_l
  Constant_x_l_ac055 : Constant  Value=x_l
  Constant_x_l_b52e5 : Constant  Value=x_l
  Constant_x_qd_67319 : Constant  Value=x_qd
  Constant_x_qd_a8925 : Constant  Value=x_qd
  Constant_x_qd_d7338 : Constant  Value=x_qd
  Constant_x_qdd_2de80 : Constant  Value=x_qdd
  Constant_x_qdd_408b6 : Constant  Value=x_qdd
  Constant_x_qdd_67a76 : Constant  Value=x_qdd
  Divide_167d4 : Product  Inputs=*/
  Divide_1b82c : Product  Inputs=*/
  Divide_47dd3 : Product  Inputs=*/
  Divide_9b124 : Product  Inputs=*/
  Divide_a3996 : Product  Inputs=*/
  Divide_d53e8 : Product  Inputs=*/
  MathFunc_cos_01cd2 : Trigonometry  Operator=cos
  MathFunc_sin_1781d : Trigonometry
  Product_05df3 : Product
  Product_12561 : Product
  Product_4fe99 : Product
  Product_52b2a : Product
  Product_7b14f : Product
  Product_81acd : Product
  Product_aaa91 : Product
  Product_d1d8e : Product
  Product_fa3b3 : Product
  Product_fbed1 : Product
  Product_ffb25 : Product
  Subtract_0ac1d : Sum  Inputs=+-
  Subtract_25275 : Sum  Inputs=+-
  Subtract_28c87 : Sum  Inputs=+-
  Subtract_38b1e : Sum  Inputs=+-
  Subtract_5ccbb : Sum  Inputs=+-
  Subtract_7341b : Sum  Inputs=+-
  Subtract_adf13 : Sum  Inputs=+-
  Subtract_e53bc : Sum  Inputs=+-
  Blockout_i_d_SG_D_3_2136b : Outport
  wires:
  Constant_x_qd_67319/1 -> Subtract_adf13/1
  Subtract_28c87/1 -> Blockout_i_d_SG_D_3_2136b/1
  Constant_-1_23574/1 -> Product_81acd/1
  Constant_x_l_79434/1 -> Product_12561/2
  Constant_x_qdd_67a76/1 -> Add_ea115/2
  Constant_x_qdd_2de80/1 -> Subtract_adf13/2
  Constant_x_l_4d31d/1 -> Product_81acd/2
  Divide_47dd3/1 -> Subtract_28c87/1
  Product_81acd/1 -> Add_ea115/1
  Constant_x_ddd_9648b/1 -> Subtract_0ac1d/2
  Constant_-1_75f1e/1 -> Product_12561/1
  Constant_-1_687e4/1 -> Product_d1d8e/1
  Constant_x_l_b52e5/1 -> Product_d1d8e/2
  State_psi_1d_SG_D_3_e063f/1 -> Product_ffb25/2
  State_psi_gq_SG_D_3_033c6/1 -> Product_fa3b3/1
  Product_ffb25/1 -> Product_4fe99/1
  Add_ea115/1 -> Product_fa3b3/2
  Product_12561/1 -> Add_8a214/1
  Constant_x_qd_d7338/1 -> Add_8a214/2
  State_psi_kq_SG_D_3_67dcb/1 -> Product_fbed1/1
  Subtract_5ccbb/1 -> Divide_9b124/2
  Subtract_adf13/1 -> Product_fbed1/2
  Product_d1d8e/1 -> Add_a17fd/1
  Constant_x_ddd_259c8/1 -> Subtract_7341b/1
  Constant_x_qd_a8925/1 -> Add_a17fd/2
  Constant_-1_6883c/1 -> Product_ffb25/1
  Constant_x_dd_eff09/1 -> Subtract_0ac1d/1
  Product_fa3b3/1 -> Divide_a3996/1
  Add_8a214/1 -> Divide_a3996/2
  Product_fbed1/1 -> Divide_167d4/1
  Add_a17fd/1 -> Divide_167d4/2
  Divide_9b124/1 -> Subtract_e53bc/2
  Subtract_0ac1d/1 -> Product_4fe99/2
  State_theta_SG_D_3_0b2a8/1 -> MathFunc_cos_01cd2/1
  Constant_x_dd_b5763/1 -> Subtract_25275/1
  Product_05df3/1 -> Product_52b2a/1
  Constant_x_l_ac055/1 -> Subtract_25275/2
  Add_92cd6/1 -> Subtract_e53bc/1
  Constant_x_l_9e4c3/1 -> Subtract_7341b/2
  State_theta_SG_D_3_6b34c/1 -> MathFunc_sin_1781d/1
  Divide_a3996/1 -> Subtract_38b1e/1
  Add_dfa2f/1 -> Product_05df3/2
  Divide_167d4/1 -> Subtract_38b1e/2
  Product_4fe99/1 -> Divide_1b82c/1
  Subtract_25275/1 -> Divide_1b82c/2
  State_psi_fd_SG_D_3_2fd40/1 -> Product_7b14f/1
  Divide_d53e8/1 -> Subtract_28c87/2
  Subtract_7341b/1 -> Product_7b14f/2
  Constant_x_dd_7bc64/1 -> Subtract_5ccbb/1
  Subtract_38b1e/1 -> Add_dfa2f/1
  Constant_x_l_6f196/1 -> Subtract_5ccbb/2
  Constant_-1_cf294/1 -> Product_05df3/1
  State_psi_q_SG_D_3_1df08/1 -> Add_dfa2f/2
  Divide_1b82c/1 -> Add_92cd6/1
  State_psi_d_SG_D_3_e7225/1 -> Add_92cd6/2
  Product_7b14f/1 -> Divide_9b124/1
  MathFunc_cos_01cd2/1 -> Product_52b2a/2
  MathFunc_sin_1781d/1 -> Product_aaa91/2
  Subtract_e53bc/1 -> Product_aaa91/1
  Product_52b2a/1 -> Divide_47dd3/1
  Constant_x_qdd_408b6/1 -> Divide_47dd3/2
  Product_aaa91/1 -> Divide_d53e8/1
  Constant_x_ddd_23990/1 -> Divide_d53e8/2
